simulink model "eqns_motion_mdl_439"  (R2018b)
settings: Solver=VariableStepAuto  StartTime=0.0  StopTime=250  FixedStep=0.1  RelTol=1e-4
values from neighbouring files (symbols this model uses):
  air_data = load('air_data.csv')    [eqns_motion_script.m]    (also in eqns_motion_script_439.m)
  alpha_data = load('alpha_data.csv')    [Test_Runs_Arthur_Function.m]    (also in eqns_motion_script.m; eqns_motion_script_439.m)
  AR = De^2/Dt^2    (= 7.35623218146)    [Test_Runs_Arthur_Function.m]    (also in engineMass.m = engine.output.eql.aeat(3); eqns_motion_script.m = 7.52170654272; eqns_motion_script_439.m = 7.52170654272)
  At = pi*Dt^2/4    (= 7.87496924005)    [Test_Runs_Arthur_Function.m]    (also in engineMass.m = cstar*mdot/(Pc*g); eqns_motion_script.m = 7.53210209316; eqns_motion_script_439.m = 7.53210209316)
  burn_time = (200000+Impulse_Savings)/Thrust    [One_Run.m]    (also in Purdue_Setup.m = 40; Setup.m = 42; Test_Runs.m = 40; Test_Runs_Arthur_Function.m = 39.2156862745)
  Cd_data = load('cd_M.csv')    [Test_Runs_Arthur_Function.m]    (also in eqns_motion_script.m; eqns_motion_script_439.m)
  CG = CG + CG_dot*ts    (= 2.21669239668)    [attempt2.m]    (also in eqns_motion_script.m = 3.6576; eqns_motion_script_439.m = 3.6576; flight_controller.m; flight_sim_3D.m)
  Cn_data = load('cl_M_a.csv')    [Test_Runs_Arthur_Function.m]    (also in eqns_motion_script.m; eqns_motion_script_439.m)
  cp = [CP-CG; 0; 0]    [Y_eqns.m]    (also in Z_eqns.m; attempt2.m; eqns_motion_script.m = 910; eqns_motion_script_439.m = 910)
  Cp_data = load('cp_M_a.csv')    [Test_Runs_Arthur_Function.m]    (also in eqns_motion_script.m; eqns_motion_script_439.m)
  d = D * -v_unit    [Y_eqns.m]    (also in Z_eqns.m; attempt2.m; eqns_motion_script.m = 0.4064; eqns_motion_script_439.m = 0.4064)
  day = 119    [eqns_motion_script.m]    (also in eqns_motion_script_439.m)
  De = 8.5883    [Test_Runs_Arthur_Function.m]    (also in engineMass.m = sqrt(4*Ae/pi); eqns_motion_script.m = 8.4932; eqns_motion_script_439.m = 8.4932)
  h0 = 4595*0.3048    (= 1400.556)    [eqns_motion_script.m]    (also in eqns_motion_script_439.m)
  h_trailer = 75*0.3048    (= 22.86)    [eqns_motion_script.m]    (also in eqns_motion_script_439.m)
  k_he = 0.1177    [eqns_motion_script.m]    (also in eqns_motion_script_439.m)
  kc = 0.35    [eqns_motion_script.m]    (also in eqns_motion_script_439.m)
  lat = 32.9861    [eqns_motion_script.m]    (also in eqns_motion_script_439.m)
  len = 24*0.3048    (= 7.3152)    [attempt2.m]    (also in eqns_motion_script.m; eqns_motion_script_439.m; flight_controller.m; flight_sim_3D.m)
  lon = -106.9717    [eqns_motion_script.m]    (also in eqns_motion_script_439.m)
  M_data = load('M_data.csv')    [Test_Runs_Arthur_Function.m]    (also in eqns_motion_script.m; eqns_motion_script_439.m)
  m_dry = m_dry_lbm / 2.20462    (= 34.0194682077)    [SIM_1DOF.m]    (also in attempt2.m = 330.474171429; eqns_motion_script.m = 291.222339948; eqns_motion_script_439.m = 291.222339948; flight_controller.m = 330.474171429)
  m_wet = 1300*0.453592    (= 589.6696)    [attempt2.m]    (also in eqns_motion_script.m = 679.17690936; eqns_motion_script_439.m = 679.17690936; flight_controller.m; flight_sim_3D.m)
  material_density = 2700    [eqns_motion_script.m]    (also in eqns_motion_script_439.m)
  mdot = mdot + mdot_ffc    [engineMass.m]    (also in eqns_motion_script.m = 10.58683728; eqns_motion_script_439.m = 10.58683728)
  mdot_th = mdot*throttle    (= 10.58683728)    [eqns_motion_script.m]    (also in eqns_motion_script_439.m)
  mu = 1.512041288*(Talt^(3/2))/(Talt+120)    (= 18.1205671028)    [altcond.m]    (also in altcond1.m = 1.512041288*(Talt^(3/2))/(Talt+120); altcond2.m = 1.512041288*(Talt^(3/2))/(Talt+120); eqns_motion_script.m = 0.42; eqns_motion_script_439.m = 0.42)
  Pc = 450    [Test_Runs_Arthur_Function.m]    (also in eqns_motion_script.m; eqns_motion_script_439.m)
  Pe = pressure_integral(end)/burn_time    [Test_Runs.m]    (also in Test_Runs_Arthur_Function.m = 10; eqns_motion_script.m = 10; eqns_motion_script_439.m = 10)
  psi0 = 0    [eqns_motion_script.m]    (also in eqns_motion_script_439.m)
  r = diam/2    (= 0.2286)    [attempt2.m]    (also in eqns_motion_script.m = 0.2032; eqns_motion_script_439.m = 0.2032; flight_controller.m; flight_sim_3D.m)
  sec = 12*3600    (= 43200)    [eqns_motion_script.m]    (also in eqns_motion_script_439.m)
  T = torque_total * 0.113    [PumpSizingModel.m]    (also in attempt2.m = 7000; eqns_motion_script.m = 5100; eqns_motion_script_439.m = 5100; flight_controller.m = 7000)
  t_th = 0    [eqns_motion_script.m]    (also in eqns_motion_script_439.m)
  T_th = T*throttle    (= 5100)    [eqns_motion_script.m]    (also in eqns_motion_script_439.m)
  tc = 0.000    (= 0)    [eqns_motion_script.m]    (also in eqns_motion_script_439.m)
  theta0 = 0    [eqns_motion_script.m]    (also in eqns_motion_script_439.m)
  u0 = 0.1    [eqns_motion_script.m]    (also in eqns_motion_script_439.m)
  v0 = 0.0    (= 0)    [eqns_motion_script.m]    (also in eqns_motion_script_439.m)
  w0 = 0.0    (= 0)    [eqns_motion_script.m]    (also in eqns_motion_script_439.m)
  x = CEA('problem','rocket','equilibrium','o/f', linspace(1,2,5),'p,Mpa',4,'reactants','fuel','N2H4(L)','wt    [CEA.m]    (also in Test_Runs_Arthur_Function.m = 2; eqns_motion_script.m = 0.1; eqns_motion_script_439.m = 0.1; getContour.m = [x_chamber(1:end-1) fliplr(Cx_parabola) x_1_5(2:end) x_0_4(2)
  x1 = len*3/4    (= 5.4864)    [eqns_motion_script.m]    (also in eqns_motion_script_439.m)
libraries: vrlib x8, simulink_extras x6, aerolibutil x3, sharedtransform x2, aerolibasang x2, aerolibconvert2 x2, aerolibatmos2 x1, aerolibadyn x1, aerolibanimutils x1, sharedutil x1, aerolibwind2 x1
settings Model: Creator=Arthur de Waleffe  LastModifiedBy=bartk

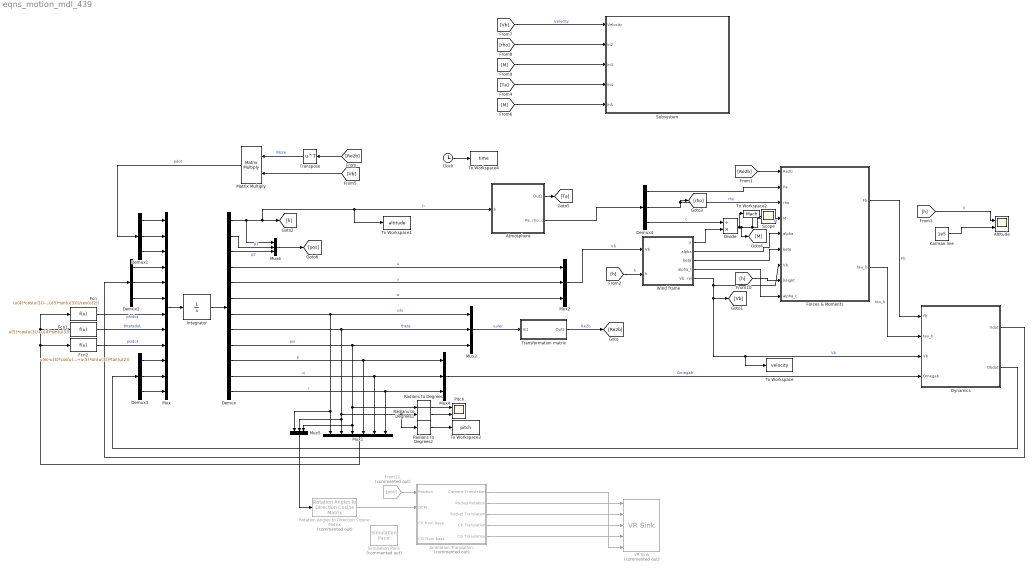
== system eqns_motion_mdl_439 ==
  Altitude : Scope  NumInputPorts=2
  Animation Translation : Subsystem  Commented=on
  Atmosphere : Subsystem
  Clock : Clock
  Demux : Demux  Outputs=12
  Demux{1..4} (4 alike) : Demux  Outputs=3
  Divide : Product  Inputs=/*
  Dynamics : Subsystem
  Fcn : Fcn  Expr=(u(4)*cos(u(3))-u(5)*sin(u(3)))/cos(u(2))
  Fcn1 : Fcn  Expr=u(5)*cos(u(3))+u(4)*sin(u(3))
  Fcn2 : Fcn  Expr=u(6)-u(4)*cos(u(3))*tan(u(2))+u(5)*sin(u(3))*tan(u(2))
  Forces & Moments : Subsystem
  From11 : From  Commented=on  GotoTag=pos
  Integrator : Integrator  InitialCondition=[h0;0;0;u0;v0;w0;0;theta0;psi0;0;0;0]
  Karman line : Constant  Value=1e5
  Matrix Multiply : Product  Multiplication=Matrix(*)
  Mux : Mux  Inputs=12
  Mux1 : Mux  Inputs=6
  Mux{2..6} (5 alike) : Mux  Inputs=3
  Pitch : Scope  NumInputPorts=2
  Radians to Degrees : simulink_extras/Transformations/Radians to Degrees
  Radians to Degrees1 : simulink_extras/Transformations/Radians to Degrees
  Radians to Degrees2 : simulink_extras/Transformations/Radians to Degrees
  Rotation Angles to Direction Cosine Matrix : sharedtransform/Rotation Angles to Direction Cosine Matrix  Commented=on  rotationOrder=ZYX  aMode=aMode
      settings: SourceProductBaseCode=AE
  Scope : Scope
  Simulation Pace : aerolibanimutils/Simulation Pace  Commented=on  SimulationPace=1  SleepMode=Auto  OutputPaceError=off  SampleTime=1/30
  Subsystem : Subsystem
  To Workspace : ToWorkspace  VariableName=velocity  SampleTime=-1
  To Workspace1 : ToWorkspace  VariableName=altitude  SampleTime=-1
  To Workspace2 : ToWorkspace  VariableName=Mach  SaveFormat=Timeseries  SampleTime=-1
  To Workspace3 : ToWorkspace  VariableName=pitch  SaveFormat=Timeseries  SampleTime=-1
  To Workspace4 : ToWorkspace  VariableName=time  SampleTime=-1
  Transformation matrix : Subsystem
  Transpose : Math  Operator=transpose  SaturateOnIntegerOverflow=on
  VR Sink : vrlib/VR Sink  Commented=on  InstantiateOnLoad=on  SampleTime=0.1  ViewEnable=on  RemoteChange=off  RemoteView=off  FieldsWritten=Rocket.rotation.4.1.1.double#Rocket.translation.3.1.1.double#CP.translation.3.1.1.double#CG.translation.3.1.1.double#Camera.position.3.1.1.double  WorldFileName=liftoff.WRL  AutoView=off  VideoDimensions=[]  AllowVariableSize=off
      settings: SourceProductBaseCode=VR
  "Wind frame " : Subsystem
  wires:
  Integrator/1 -> Demux/1
  Mux/1 -> Integrator/1
  Demux/4 -> Mux2/1  "u"
  Demux/5 -> Mux2/2  "v"
  Demux/6 -> Mux2/3  "w"
  Demux/7 -> Mux3/1, Mux5/1, Mux1/1  "phi"
  Demux/8 -> Mux3/2, Radians to Degrees2/1, Radians to Degrees1/1, Mux5/2, Mux1/2  "theta"
  Demux/9 -> Mux3/3, Mux5/3, Mux1/3, Radians to Degrees/1  "psi"
  Demux/10 -> Mux4/1, Mux1/4  "p"
  Demux/12 -> Mux4/3, Mux1/6  "r"
  Demux/11 -> Mux4/2, Mux1/5  "q"
  Fcn/1 -> Mux/7  "phidot"
  Fcn1/1 -> Mux/8  "thtetadot"
  Fcn2/1 -> Mux/9  "psidot"
  Mux1/1 -> Fcn2/1, Fcn/1, Fcn1/1
  Mux3/1 -> Transformation matrix/1(In1)  "euler"
  Transpose/1 -> Matrix Multiply/1  "Rb2e"
  Matrix Multiply/1 -> Demux1/1  "pdot"
  Demux1/2 -> Mux/2
  Demux1/1 -> Mux/1
  Demux1/3 -> Mux/3
  Demux2/1 -> Mux/4
  Demux2/2 -> Mux/5
  Demux2/3 -> Mux/6
  Demux4/2 -> [rho], Forces & Moments/3(rho)  "rho"
  Demux3/1 -> Mux/10
  Demux3/2 -> Mux/11
  Demux3/3 -> Mux/12
  Demux4/3 -> Divide/1  "c"
  Divide/1 -> To Workspace2/1, [M], Scope/1, Forces & Moments/4(M)  "M"
  "Wind frame "/1(V) -> Divide/2
  "Wind frame "/2(alpha) -> Forces & Moments/5(alpha)
  "Wind frame "/3(beta) -> Forces & Moments/6(beta)
  "Wind frame "/4(alpha_t) -> Forces & Moments/9(alpha_t)
  Demux/2 -> Mux6/2  "p1"
  Demux/3 -> Mux6/3  "p2"
  Forces & Moments/1(Fb) -> Dynamics/1(Fb)  "Fb"
  Forces & Moments/2(tau_b) -> Dynamics/2(tau_b)  "tau_b"
  Mux4/1 -> Dynamics/4(Omegab)  "Omegab"
  Dynamics/1(Vdot) -> Demux2/1
  Dynamics/2(Obdot) -> Demux3/1
  Transformation matrix/1(Out1) -> [Re2b]  "Re2b"
  [Re2b] -> Transpose/1
  [Re2b] -> Forces & Moments/1(Re2b)
  [Vb] -> Matrix Multiply/2
  Karman line/1 -> Altitude/2
  [h] -> Altitude/1  "h"
  "Wind frame "/5("Vb, rel") -> [Vb], To Workspace/1, Dynamics/3(Vb), Forces & Moments/7(Vb)  "Vb"
  Mux2/1 -> "Wind frame "/1(Vb)  "Vb"
  Demux4/1 -> Forces & Moments/2(Pa)
  Atmosphere/2("Pa, rho, c") -> Demux4/1
  Demux/1 -> Mux6/1, To Workspace1/1, Atmosphere/1(h), [h]  "h"
  [h] -> "Wind frame "/2(h)  "h"
  [Ta] -> Subsystem/4(In4)
  [M] -> Subsystem/3(In3)
  [Vb] -> Subsystem/1(Velocity)  "Velocity"
  [M] -> Subsystem/5(In5)
  [rho] -> Subsystem/2(In2)
  Atmosphere/1(Out1) -> [Ta]
  [h] -> Forces & Moments/8(height)
  Animation Translation/2(Rocket Rotation) -> VR Sink/1
  Animation Translation/3(Rocket Translation) -> VR Sink/2
  Animation Translation/4(CP Translation) -> VR Sink/3
  Animation Translation/1(Camera Translation) -> VR Sink/5
  Animation Translation/5(CG Translation) -> VR Sink/4
  Mux5/1 -> Rotation Angles to Direction Cosine Matrix/1
  Rotation Angles to Direction Cosine Matrix/1 -> Animation Translation/2(DCM)
  Mux6/1 -> [pos]
  From11/1 -> Animation Translation/1(Position)
  Radians to Degrees/1 -> Pitch/1
  Radians to Degrees1/1 -> Pitch/2
  Radians to Degrees2/1 -> To Workspace3/1
  Clock/1 -> To Workspace4/1

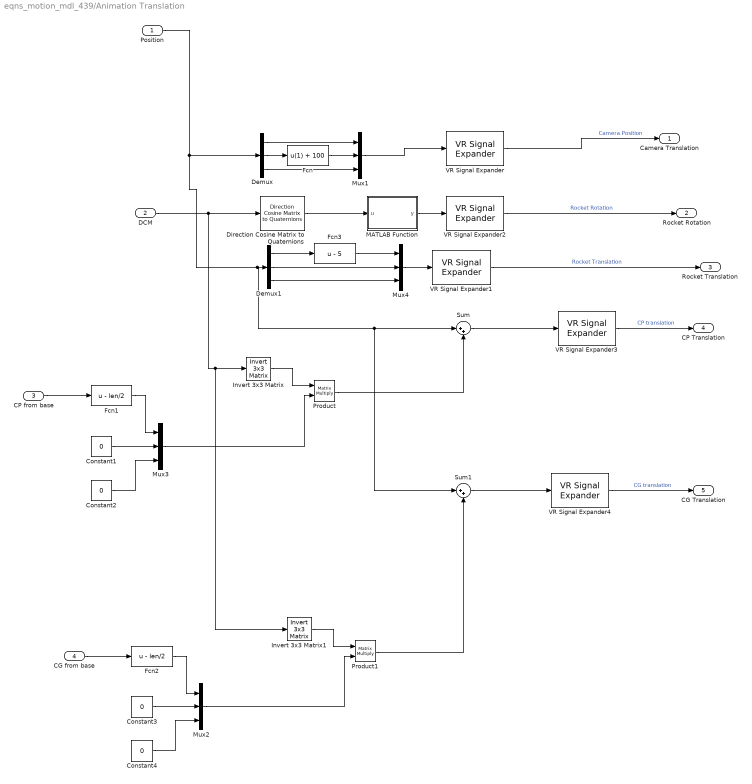
== system eqns_motion_mdl_439/Animation Translation ==
  Position : Inport
  DCM : Inport  Port=2
  CP from base : Inport  Port=3
  CG from base : Inport  Port=4
  Constant{1..4} (4 alike) : Constant  Value=0
  Demux : Demux  Outputs=3
  Demux1 : Demux  Outputs=3
  Direction Cosine Matrix to Quaternions : sharedtransform/Direction Cosine Matrix  to Quaternions  aMode=0  action=None  tolerance=eps(2)
      settings: SourceProductName=Aerospace Blockset  SourceProductBaseCode=AE
  Fcn : Fcn  Expr=u(1) + 100
  Fcn1 : Fcn  Expr=u - len/2
  Fcn2 : Fcn  Expr=u - len/2
  Fcn3 : Fcn  Expr=u - 5
  Invert 3x3 Matrix : aerolibutil/Invert  3x3 Matrix
  Invert 3x3 Matrix1 : aerolibutil/Invert  3x3 Matrix
  MATLAB Function : MATLAB Function  TreatAsAtomicUnit=on
  Mux{1..4} (4 alike) : Mux  Inputs=3
  Product : Product  Multiplication=Matrix(*)
  Product1 : Product  Multiplication=Matrix(*)
  Sum : Sum  Inputs=|++
  Sum1 : Sum  Inputs=|++
  VR Signal Expander{,1,3..4} (4 alike) : vrlib/VR Signal Expander  outwidth=3  outidx=[2 3 1]
      settings: SourceProductName=Simulink 3D Animation  SourceProductBaseCode=VR
  VR Signal Expander2 : vrlib/VR Signal Expander  outwidth=4  outidx=[2 3 1 4]
      settings: SourceProductName=Simulink 3D Animation  SourceProductBaseCode=VR
  Camera Translation : Outport
  Rocket Rotation : Outport  Port=2
  Rocket Translation : Outport  Port=3
  CP Translation : Outport  Port=4
  CG Translation : Outport  Port=5
  wires:
  Demux/2 -> Fcn/1
  Position/1 -> Demux1/1, Sum1/1, Sum/1, Demux/1
  Mux1/1 -> VR Signal Expander/1
  MATLAB Function/1(y) -> VR Signal Expander2/1
  DCM/1 -> Invert 3x3 Matrix1/1, Invert 3x3 Matrix/1, Direction Cosine Matrix to Quaternions/1
  Direction Cosine Matrix to Quaternions/1 -> MATLAB Function/1(u)
  Demux/3 -> Mux1/3
  Demux/1 -> Mux1/1
  Fcn/1 -> Mux1/2
  VR Signal Expander/1 -> Camera Translation/1  "Camera Position"
  CP from base/1 -> Fcn1/1
  VR Signal Expander3/1 -> CP Translation/1  "CP translation"
  Constant1/1 -> Mux3/2
  Fcn1/1 -> Mux3/1
  Constant2/1 -> Mux3/3
  Mux3/1 -> Product/2
  Product/1 -> Sum/2
  Invert 3x3 Matrix/1 -> Product/1
  Sum/1 -> VR Signal Expander3/1
  VR Signal Expander2/1 -> Rocket Rotation/1  "Rocket Rotation"
  VR Signal Expander1/1 -> Rocket Translation/1  "Rocket Translation"
  Constant4/1 -> Mux2/3
  Invert 3x3 Matrix1/1 -> Product1/1
  Mux2/1 -> Product1/2
  Fcn2/1 -> Mux2/1
  Constant3/1 -> Mux2/2
  CG from base/1 -> Fcn2/1
  Product1/1 -> Sum1/2
  Sum1/1 -> VR Signal Expander4/1
  VR Signal Expander4/1 -> CG Translation/1  "CG translation"
  Demux1/3 -> Mux4/3
  Demux1/2 -> Mux4/2
  Mux4/1 -> VR Signal Expander1/1
  Demux1/1 -> Fcn3/1
  Fcn3/1 -> Mux4/1

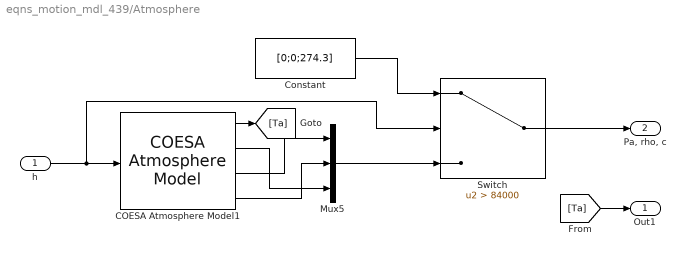
== system eqns_motion_mdl_439/Atmosphere ==
  h : Inport
  COESA Atmosphere Model1 : aerolibatmos2/COESA Atmosphere Model  units=Metric (MKS)  spec=1976 COESA-extended U.S. Standard Atmosphere  model=Profile  profile_var=High temperature  profile_percent=1%  profile_alt=5 km (16404 ft)  envelope_var=High temperature  envelope_percent=1%  action=Warning
  Constant : Constant  Value=[0;0;274.3]
  Mux5 : Mux  Inputs=3
  Switch : Switch  Criteria=u2 > Threshold  Threshold=84000
  Out1 : Outport
  "Pa, rho, c" : Outport  Port=2
  wires:
  Switch/1 -> "Pa, rho, c"/1
  COESA Atmosphere Model1/3 -> Mux5/1
  Constant/1 -> Switch/1
  Mux5/1 -> Switch/3
  COESA Atmosphere Model1/1 -> [Ta]
  COESA Atmosphere Model1/4 -> Mux5/2
  COESA Atmosphere Model1/2 -> Mux5/3
  h/1 -> COESA Atmosphere Model1/1, Switch/2
  [Ta] -> Out1/1

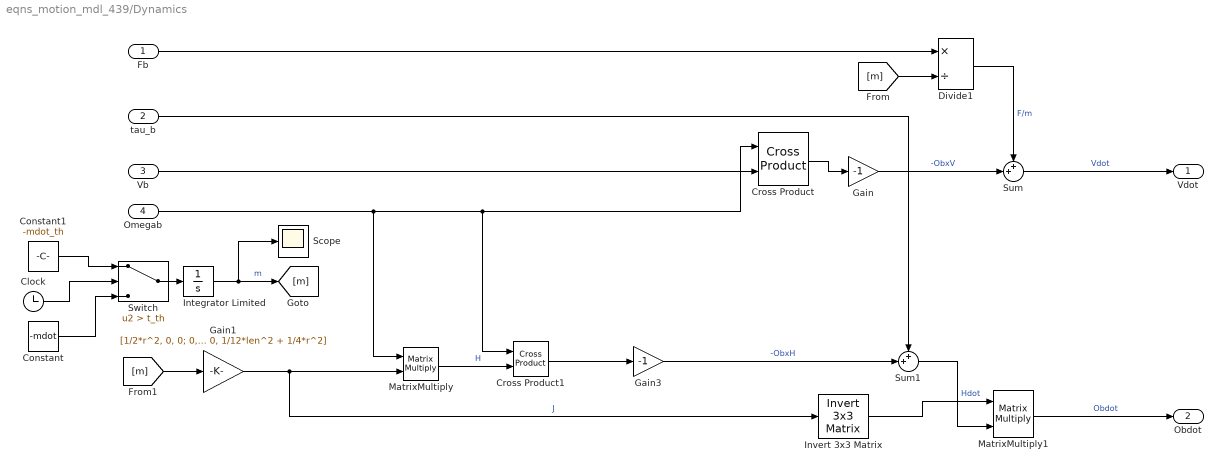
== system eqns_motion_mdl_439/Dynamics ==
  Fb : Inport
  tau_b : Inport  Port=2
  Vb : Inport  Port=3
  Omegab : Inport  Port=4
  Clock : Clock
  Constant : Constant  Value=-mdot
  Constant1 : Constant  Value=-mdot_th
  Cross Product : vrlib/Utilities/Cross Product
      settings: SourceProductBaseCode=VR
  Cross Product1 : vrlib/Utilities/Cross Product
      settings: SourceProductBaseCode=VR
  Divide1 : Product  Inputs=*/
  Gain : Gain  Gain=-1
  Gain1 : Gain  Gain=[1/2*r^2, 0, 0; 0, 1/12*len^2 + 1/4*r^2, 0; 0, 0, 1/12*len^2 + 1/4*r^2]
  Gain3 : Gain  Gain=-1
  Integrator Limited : Integrator  InitialCondition=m_wet  LimitOutput=on  UpperSaturationLimit=m_wet  LowerSaturationLimit=m_dry
  Invert 3x3 Matrix : aerolibutil/Invert  3x3 Matrix
  MatrixMultiply : Product  Multiplication=Matrix(*)
  MatrixMultiply1 : Product  Multiplication=Matrix(*)
  Scope : Scope
  Sum : Sum  Inputs=++|
  Sum1 : Sum  Inputs=++|
  Switch : Switch  Criteria=u2 > Threshold  Threshold=t_th
  Vdot : Outport
  Obdot : Outport  Port=2
  wires:
  Gain1/1 -> Invert 3x3 Matrix/1, MatrixMultiply/2  "J"
  MatrixMultiply/1 -> Cross Product1/2  "H"
  MatrixMultiply1/1 -> Obdot/1  "Obdot"
  Cross Product/1 -> Gain/1
  Sum1/1 -> MatrixMultiply1/2  "Hdot"
  Integrator Limited/1 -> Scope/1, [m]  "m"
  Gain3/1 -> Sum1/2  "-ObxH"
  Cross Product1/1 -> Gain3/1
  Omegab/1 -> Cross Product/1, Cross Product1/1, MatrixMultiply/1
  Gain/1 -> Sum/2  "-ObxV"
  Invert 3x3 Matrix/1 -> MatrixMultiply1/1
  Sum/1 -> Vdot/1  "Vdot"
  Divide1/1 -> Sum/1  "F/m"
  Vb/1 -> Cross Product/2
  Fb/1 -> Divide1/1
  tau_b/1 -> Sum1/1
  [m] -> Divide1/2
  [m] -> Gain1/1
  Clock/1 -> Switch/2
  Constant1/1 -> Switch/1
  Constant/1 -> Switch/3
  Switch/1 -> Integrator Limited/1

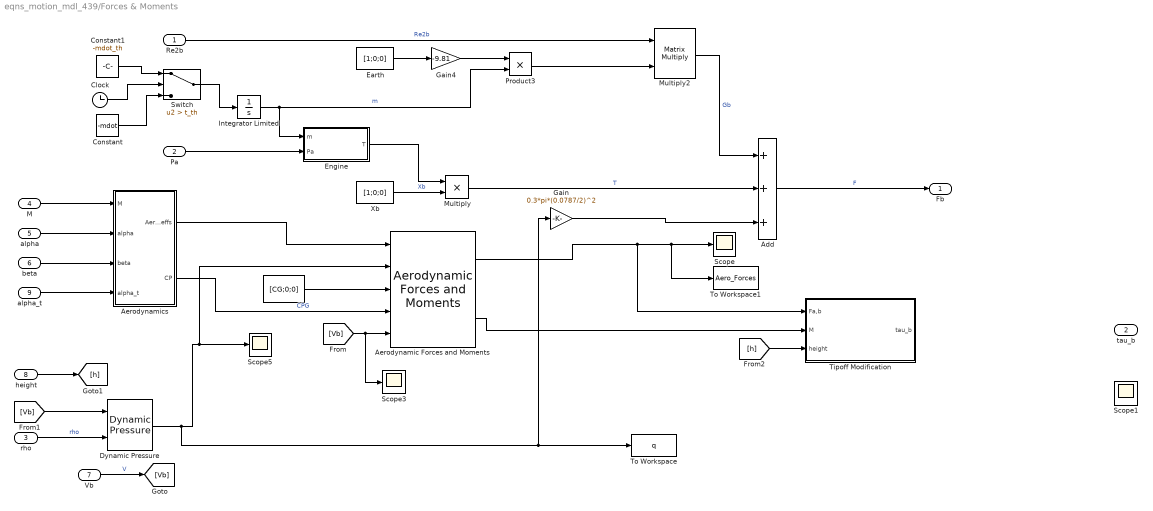
== system eqns_motion_mdl_439/Forces & Moments ==
  Re2b : Inport
  Pa : Inport  Port=2
  rho : Inport  Port=3
  M : Inport  Port=4
  alpha : Inport  Port=5
  beta : Inport  Port=6
  Vb : Inport  Port=7
  height : Inport  Port=8
  alpha_t : Inport  Port=9
  " " : Constant  Value=[CG;0;0]
  Add : Sum  Inputs=+++
  "Aerodynamic Forces and Moments " : aerolibadyn/Aerodynamic Forces and Moments   inputAxes=Wind  outputForceAxes=Body  outputMomentAxes=Body  S=S  b=d  cbar=len
      settings: SourceProductName=Aerospace Blockset
  Aerodynamics : Subsystem
  Clock : Clock
  Constant : Constant  Value=-mdot
  Constant1 : Constant  Value=-mdot_th
  Dynamic Pressure : aerolibasang/Dynamic Pressure
  Earth : Constant  Value=[1;0;0]
  Engine : Subsystem
  Gain : Gain  Gain=0.3*pi*(0.0787/2)^2
  Gain4 : Gain  Gain=-9.81
  Integrator Limited : Integrator  InitialCondition=m_wet  LimitOutput=on  UpperSaturationLimit=m_wet  LowerSaturationLimit=m_dry
  Multiply : Product
  Multiply2 : Product  Multiplication=Matrix(*)
  Product3 : Product
  Scope{,1,3,5} (4 alike) : Scope
  Switch : Switch  Criteria=u2 > Threshold  Threshold=t_th
  Tipoff Modification : Subsystem
  To Workspace : ToWorkspace  VariableName=q  SaveFormat=Timeseries  SampleTime=-1
  To Workspace1 : ToWorkspace  VariableName=Aero_Forces  SaveFormat=Timeseries  SampleTime=-1
  Xb : Constant  Value=[1;0;0]
  Fb : Outport
  tau_b : Outport  Port=2
  wires:
  Multiply2/1 -> Add/1  "Gb"
  Re2b/1 -> Multiply2/1  "Re2b"
  Earth/1 -> Gain4/1
  Add/1 -> Fb/1  "F"
  Gain4/1 -> Product3/1
  Integrator Limited/1 -> Engine/1(m), Product3/2  "m"
  Product3/1 -> Multiply2/2
  Xb/1 -> Multiply/2  "Xb"
  Multiply/1 -> Add/2  "T"
  rho/1 -> Dynamic Pressure/2  "rho"
  Aerodynamics/1(Aero coeffs) -> "Aerodynamic Forces and Moments "/1
  Aerodynamics/2(CP) -> "Aerodynamic Forces and Moments "/4  "CPG"
  " "/1 -> "Aerodynamic Forces and Moments "/3
  [Vb] -> Scope3/1, "Aerodynamic Forces and Moments "/5
  [Vb] -> Dynamic Pressure/1
  Pa/1 -> Engine/2(Pa)
  Engine/1(T) -> Multiply/1
  Switch/1 -> Integrator Limited/1
  Constant/1 -> Switch/3
  Constant1/1 -> Switch/1
  Clock/1 -> Switch/2
  [h] -> Tipoff Modification/3(height)
  "Aerodynamic Forces and Moments "/2 -> Tipoff Modification/2(M)
  "Aerodynamic Forces and Moments "/1 -> Tipoff Modification/1(Fa,b), To Workspace1/1, Scope/1
  height/1 -> [h]
  Vb/1 -> [Vb]  "V"
  alpha/1 -> Aerodynamics/2(alpha)
  beta/1 -> Aerodynamics/3(beta)
  M/1 -> Aerodynamics/1(M)
  Dynamic Pressure/1 -> Gain/1, To Workspace/1, Scope5/1, "Aerodynamic Forces and Moments "/2
  alpha_t/1 -> Aerodynamics/4(alpha_t)
  Gain/1 -> Add/3

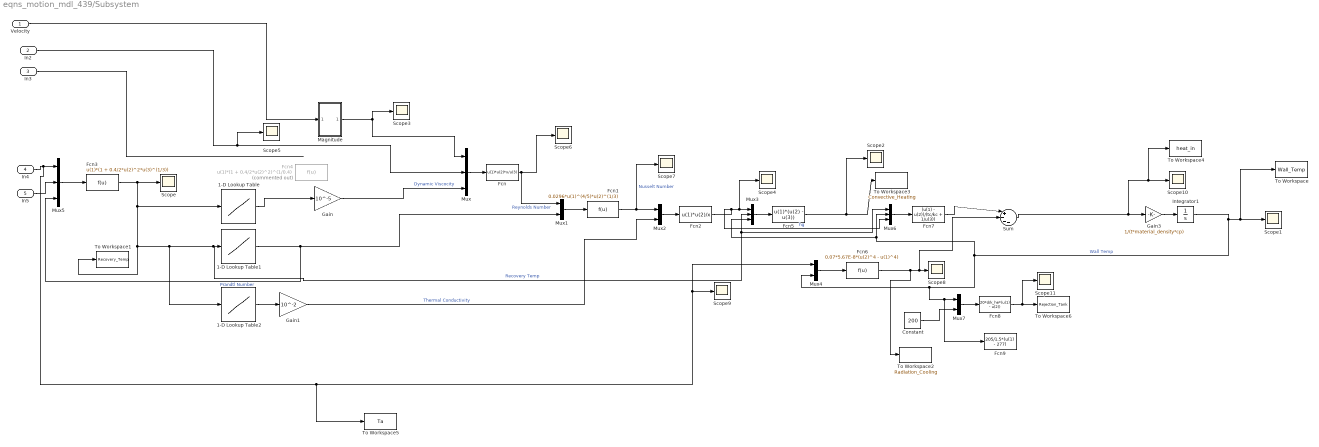
== system eqns_motion_mdl_439/Subsystem ==
  Velocity : Inport
  In2 : Inport  Port=2
  In3 : Inport  Port=3
  In4 : Inport  Port=4
  In5 : Inport  Port=5
  1-D Lookup Table : Lookup_n-D  NumberOfTableDimensions=1  BreakpointsForDimension1=air_data(:,1)  Table=air_data(:,5)  InternalRulePriority=Speed  RndMeth=Simplest  InputSameDT=on
  1-D Lookup Table1 : Lookup_n-D  NumberOfTableDimensions=1  BreakpointsForDimension1=air_data(:,1)  Table=air_data(:,7)  InternalRulePriority=Speed  RndMeth=Simplest  InputSameDT=on
  1-D Lookup Table2 : Lookup_n-D  NumberOfTableDimensions=1  BreakpointsForDimension1=air_data(:,1)  Table=air_data(:,6)  InternalRulePriority=Speed  RndMeth=Simplest  InputSameDT=on
  Constant : Constant  Value=200
  Fcn : Fcn  Expr=u(1)*u(2)*x/u(3)
  Fcn1 : Fcn  Expr=0.0296*u(1)^(4/5)*u(2)^(1/3)
  Fcn2 : Fcn  Expr=u(1)*u(2)/x
  Fcn3 : Fcn  Expr=u(1)*(1 + 0.4/2*u(2)^2*u(3)^(1/3))
  Fcn4 : Fcn  Commented=on  Expr=u(1)*(1 + 0.4/2*u(2)^2)^(1/0.4)
  Fcn5 : Fcn  Expr=u(1)*(u(2) - u(3))
  Fcn6 : Fcn  Expr=0.07*5.67E-8*(u(2)^4 - u(1)^4)
  Fcn7 : Fcn  Expr=(u(1) - u(2))/(tc/kc + 1/u(3))
  Fcn8 : Fcn  Expr=20*d/k_he*(u(1) - u(2))
  Fcn9 : Fcn  Expr=205/1.5*(u(1) - 277)
  Gain : Gain  Gain=10^-5
  Gain1 : Gain  Gain=10^-2
  Gain3 : Gain  Gain=1/(t*material_density*cp)
  Integrator1 : Integrator  InitialCondition=277
  Magnitude : Subsystem
  Mux{,3,5..6} (4 alike) : Mux  Inputs=3
  Mux{1..2,4,7} (4 alike) : Mux  Inputs=2
  Scope{,1..11} (12 alike) : Scope
  Sum : Sum  Inputs=|+---
  To Workspace : ToWorkspace  VariableName=Wall_Temp  SaveFormat=Timeseries  SampleTime=-1
  To Workspace1 : ToWorkspace  VariableName=Recovery_Temp  SaveFormat=Timeseries  SampleTime=-1
  To Workspace2 : ToWorkspace  VariableName=Radiation_Cooling  SaveFormat=Timeseries  SampleTime=-1
  To Workspace3 : ToWorkspace  VariableName=Convective_Heating  SaveFormat=Timeseries  SampleTime=-1
  To Workspace4 : ToWorkspace  VariableName=heat_in  SaveFormat=Structure With Time  SampleTime=-1
  To Workspace5 : ToWorkspace  VariableName=Ta  SaveFormat=Timeseries  SampleTime=-1
  To Workspace6 : ToWorkspace  VariableName=Rejection_Tank  SaveFormat=Timeseries  SampleTime=-1
  wires:
  Gain1/1 -> Mux2/2  "Thermal Conductivity"
  Mux5/1 -> Fcn3/1
  Fcn3/1 -> To Workspace1/1, 1-D Lookup Table2/1, Mux6/1, Mux3/2, 1-D Lookup Table1/1, 1-D Lookup Table/1, Scope/1  "Recovery Temp"
  1-D Lookup Table1/1 -> Mux1/2, Mux5/3  "Prandtl Number"
  In2/1 -> Mux/2, Scope5/1
  In3/1 -> ?
  1-D Lookup Table2/1 -> Gain1/1
  Gain/1 -> Mux/3  "Dynamic Viscocity"
  Integrator1/1 -> Mux6/2, Mux3/3, Fcn9/1, Mux7/1, Mux4/2, To Workspace/1, Scope1/1  "Wall Temp"
  In5/1 -> Mux5/2
  Magnitude/1(Out1) -> Mux/1, Scope3/1
  1-D Lookup Table/1 -> Gain/1
  Velocity/1 -> Magnitude/1(Velocity)
  In4/1 -> To Workspace5/1, Scope9/1, Mux4/1, Mux5/1
  Mux/1 -> Fcn/1
  Fcn/1 -> Mux1/1, Scope6/1  "Reynolds Number"
  Mux1/1 -> Fcn1/1
  Fcn1/1 -> Scope7/1, Mux2/1  "Nusselt Number"
  Mux2/1 -> Fcn2/1
  Fcn2/1 -> Scope4/1, Mux3/1, Mux6/3  "hg"
  Mux3/1 -> Fcn5/1
  Fcn5/1 -> Scope2/1, To Workspace3/1
  Fcn6/1 -> To Workspace2/1, Sum/2, Scope8/1
  Mux4/1 -> Fcn6/1
  Gain3/1 -> Integrator1/1
  Fcn7/1 -> Sum/1
  Mux6/1 -> Fcn7/1
  Constant/1 -> Mux7/2
  Mux7/1 -> Fcn8/1
  Fcn8/1 -> Scope11/1, To Workspace6/1
  Sum/1 -> To Workspace4/1, Scope10/1, Gain3/1

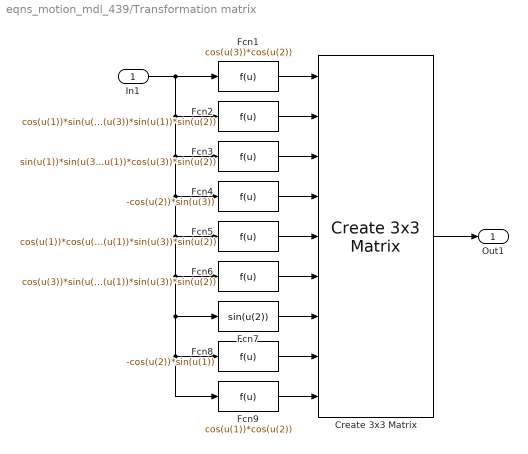
== system eqns_motion_mdl_439/Transformation matrix ==
  In1 : Inport
  Create 3x3 Matrix : sharedutil/Create 3x3 Matrix  aMode=aMode
  Fcn1 : Fcn  Expr=cos(u(3))*cos(u(2))
  Fcn2 : Fcn  Expr=cos(u(1))*sin(u(3)) + cos(u(3))*sin(u(1))*sin(u(2))
  Fcn3 : Fcn  Expr=sin(u(1))*sin(u(3)) - cos(u(1))*cos(u(3))*sin(u(2))
  Fcn4 : Fcn  Expr=-cos(u(2))*sin(u(3))
  Fcn5 : Fcn  Expr=cos(u(1))*cos(u(3)) - sin(u(1))*sin(u(3))*sin(u(2))
  Fcn6 : Fcn  Expr=cos(u(3))*sin(u(1)) + cos(u(1))*sin(u(3))*sin(u(2))
  Fcn7 : Fcn  Expr=sin(u(2))
  Fcn8 : Fcn  Expr=-cos(u(2))*sin(u(1))
  Fcn9 : Fcn  Expr=cos(u(1))*cos(u(2))
  Out1 : Outport
  wires:
  In1/1 -> Fcn9/1, Fcn8/1, Fcn7/1, Fcn6/1, Fcn5/1, Fcn4/1, Fcn3/1, Fcn2/1, Fcn1/1
  Fcn9/1 -> Create 3x3 Matrix/9
  Fcn8/1 -> Create 3x3 Matrix/8
  Fcn7/1 -> Create 3x3 Matrix/7
  Fcn6/1 -> Create 3x3 Matrix/6
  Fcn5/1 -> Create 3x3 Matrix/5
  Fcn4/1 -> Create 3x3 Matrix/4
  Fcn3/1 -> Create 3x3 Matrix/3
  Fcn2/1 -> Create 3x3 Matrix/2
  Fcn1/1 -> Create 3x3 Matrix/1
  Create 3x3 Matrix/1 -> Out1/1

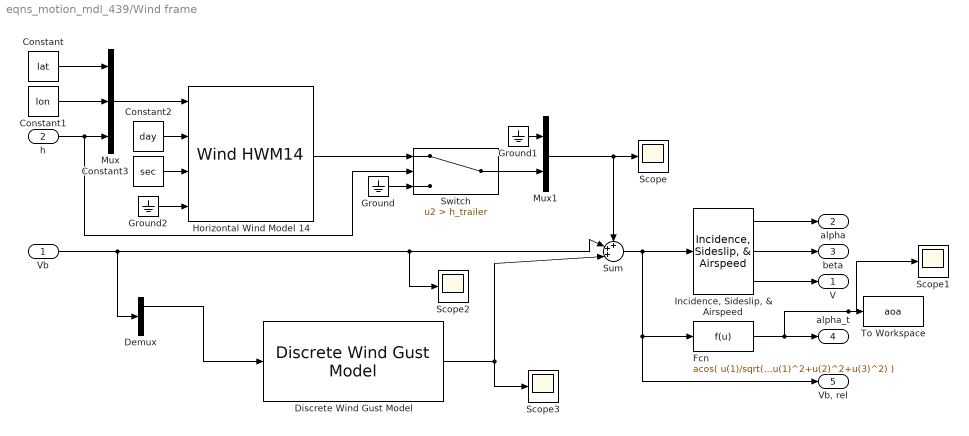
== system eqns_motion_mdl_439/Wind frame  ==
  Vb : Inport
  h : Inport  Port=2
  Constant : Constant  Value=lat
  Constant1 : Constant  Value=lon
  Constant2 : Constant  Value=day
  Constant3 : Constant  Value=sec
  Demux : Demux  Outputs=3
  Discrete Wind Gust Model : aerolibwind2/Discrete Wind Gust Model  units=Metric (MKS)  Gx=on  Gy=on  Gz=on  t_0=20  d_m=[100 100 100]  v_m=[0 0 0]
      settings: SourceProductName=Aerospace Blockset
  Fcn : Fcn  Expr=acos( u(1)/sqrt(u(1)^2+u(2)^2+u(3)^2) )
  Ground : Ground
  Ground1 : Ground
  Ground2 : Ground
  Horizontal Wind Model 14 : WindHWM14  model=Total
  "Incidence, Sideslip, & Airspeed" : aerolibasang/Incidence, Sideslip, & Airspeed
      settings: SourceProductName=Aerospace Blockset
  Mux : Mux  Inputs=3
  Mux1 : Mux  Inputs=2
  Scope{,1..3} (4 alike) : Scope
  Sum : Sum  Inputs=+++|
  Switch : Switch  Criteria=u2 > Threshold  Threshold=h_trailer
  To Workspace : ToWorkspace  VariableName=aoa  SaveFormat=Timeseries  SampleTime=-1
  V : Outport
  alpha : Outport  Port=2
  beta : Outport  Port=3
  alpha_t : Outport  Port=4
  "Vb, rel" : Outport  Port=5
  wires:
  Sum/1 -> "Vb, rel"/1, Fcn/1, "Incidence, Sideslip, & Airspeed"/1
  "Incidence, Sideslip, & Airspeed"/3 -> V/1
  "Incidence, Sideslip, & Airspeed"/1 -> alpha/1
  "Incidence, Sideslip, & Airspeed"/2 -> beta/1
  Fcn/1 -> Scope1/1, To Workspace/1, alpha_t/1
  h/1 -> Switch/2, Mux/3
  Mux/1 -> Horizontal Wind Model 14/1
  Constant1/1 -> Mux/2
  Constant/1 -> Mux/1
  Constant2/1 -> Horizontal Wind Model 14/2
  Constant3/1 -> Horizontal Wind Model 14/3
  Horizontal Wind Model 14/1 -> Switch/1
  Ground/1 -> Switch/3
  Switch/1 -> Mux1/2
  Ground1/1 -> Mux1/1
  Vb/1 -> Demux/1, Scope2/1, Sum/2
  Ground2/1 -> Horizontal Wind Model 14/4
  Mux1/1 -> Sum/1, Scope/1
  Discrete Wind Gust Model/1 -> Scope3/1, Sum/3
  Demux/1 -> Discrete Wind Gust Model/1

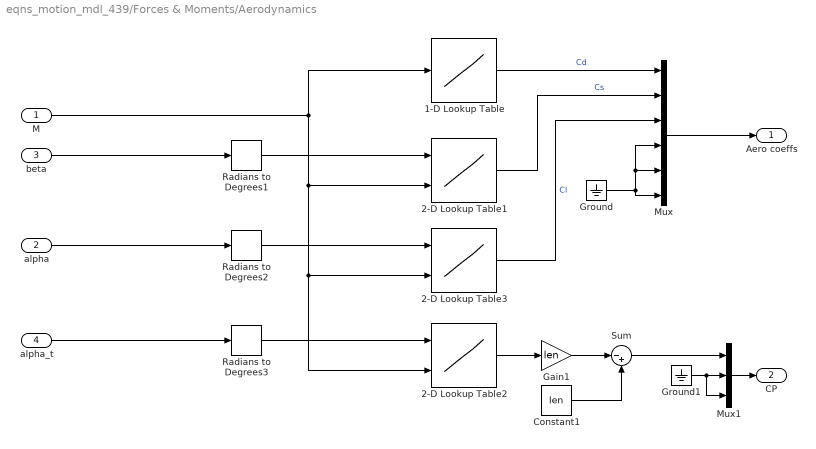
== system eqns_motion_mdl_439/Forces & Moments/Aerodynamics ==
  M : Inport
  alpha : Inport  Port=2
  beta : Inport  Port=3
  alpha_t : Inport  Port=4
  1-D Lookup Table : Lookup_n-D  NumberOfTableDimensions=1  BreakpointsForDimension1=M_data  Table=Cd_data  InternalRulePriority=Speed  RndMeth=Simplest  InputSameDT=on
  2-D Lookup Table1 : Lookup_n-D  BreakpointsForDimension1=alpha_data  BreakpointsForDimension2=M_data  Table=Cn_data  InternalRulePriority=Speed  RndMeth=Simplest  InputSameDT=on
  2-D Lookup Table2 : Lookup_n-D  BreakpointsForDimension1=alpha_data  BreakpointsForDimension2=M_data  Table=Cp_data  InternalRulePriority=Speed  RndMeth=Simplest  InputSameDT=on
  2-D Lookup Table3 : Lookup_n-D  BreakpointsForDimension1=alpha_data  BreakpointsForDimension2=M_data  Table=Cn_data  InternalRulePriority=Speed  RndMeth=Simplest  InputSameDT=on
  Constant1 : Constant  Value=len  VectorParams1D=off
  Gain1 : Gain  Gain=len
  Ground : Ground
  Ground1 : Ground
  Mux : Mux  Inputs=6
  Mux1 : Mux  Inputs=3
  Radians to Degrees1 : simulink_extras/Transformations/Radians to Degrees
  Radians to Degrees2 : simulink_extras/Transformations/Radians to Degrees
  Radians to Degrees3 : simulink_extras/Transformations/Radians to Degrees
  Sum : Sum  Inputs=|-+
  Aero coeffs : Outport
  CP : Outport  Port=2
  wires:
  1-D Lookup Table/1 -> Mux/1  "Cd"
  2-D Lookup Table2/1 -> Gain1/1
  2-D Lookup Table1/1 -> Mux/2  "Cs"
  2-D Lookup Table3/1 -> Mux/3  "Cl"
  beta/1 -> Radians to Degrees1/1
  alpha/1 -> Radians to Degrees2/1
  M/1 -> 2-D Lookup Table1/2, 2-D Lookup Table2/2, 2-D Lookup Table3/2, 1-D Lookup Table/1
  Radians to Degrees1/1 -> 2-D Lookup Table1/1
  Radians to Degrees2/1 -> 2-D Lookup Table3/1
  alpha_t/1 -> Radians to Degrees3/1
  Radians to Degrees3/1 -> 2-D Lookup Table2/1
  Ground/1 -> Mux/4, Mux/5, Mux/6
  Mux/1 -> Aero coeffs/1
  Gain1/1 -> Sum/1
  Constant1/1 -> Sum/2
  Sum/1 -> Mux1/1
  Mux1/1 -> CP/1
  Ground1/1 -> Mux1/2, Mux1/3

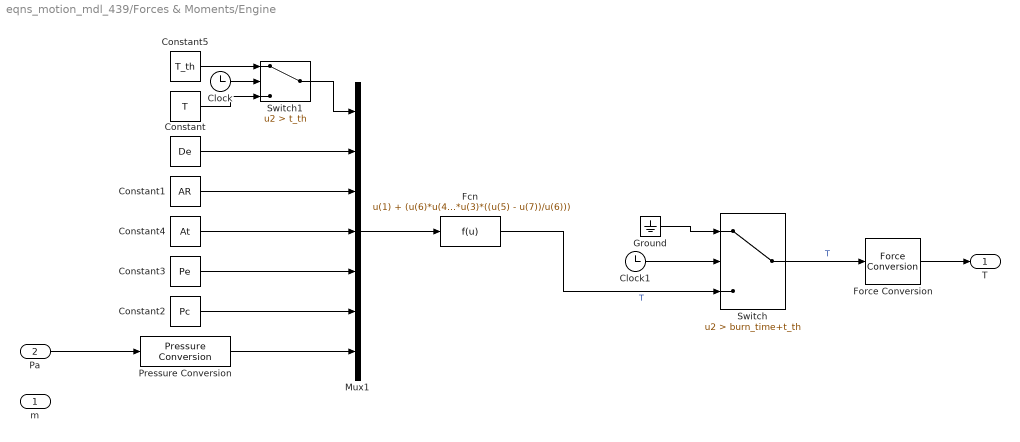
== system eqns_motion_mdl_439/Forces & Moments/Engine ==
  m : Inport
  Pa : Inport  Port=2
  " " : Constant  Value=T
  Clock : Clock
  Clock1 : Clock
  Constant : Constant  Value=De
  Constant1 : Constant  Value=AR
  Constant2 : Constant  Value=Pc
  Constant3 : Constant  Value=Pe
  Constant4 : Constant  Value=At
  Constant5 : Constant  Value=T_th
  Fcn : Fcn  Expr=u(1) + (u(6)*u(4)*u(3)*((u(5) - u(7))/u(6)))
  Force Conversion : aerolibconvert2/Force Conversion  IU=lbf  OU=N
      settings: SourceProductName=Aerospace Blockset  SourceProductBaseCode=AE
  Ground : Ground
  Mux1 : Mux  Inputs=7
  Pressure Conversion : aerolibconvert2/Pressure Conversion  IU=Pa  OU=psi
      settings: SourceProductName=Aerospace Blockset  SourceProductBaseCode=AE
  Switch : Switch  Criteria=u2 > Threshold  Threshold=burn_time+t_th
  Switch1 : Switch  Criteria=u2 > Threshold  Threshold=t_th
  T : Outport
  wires:
  Constant2/1 -> Mux1/6
  Constant3/1 -> Mux1/5
  Mux1/1 -> Fcn/1
  Constant1/1 -> Mux1/3
  Constant/1 -> Mux1/2
  Pa/1 -> Pressure Conversion/1
  Constant4/1 -> Mux1/4
  Switch/1 -> Force Conversion/1  "T"
  Force Conversion/1 -> T/1
  Pressure Conversion/1 -> Mux1/7
  Constant5/1 -> Switch1/1
  " "/1 -> Switch1/3
  Clock/1 -> Switch1/2
  Switch1/1 -> Mux1/1
  Clock1/1 -> Switch/2
  Ground/1 -> Switch/1
  Fcn/1 -> Switch/3  "T"

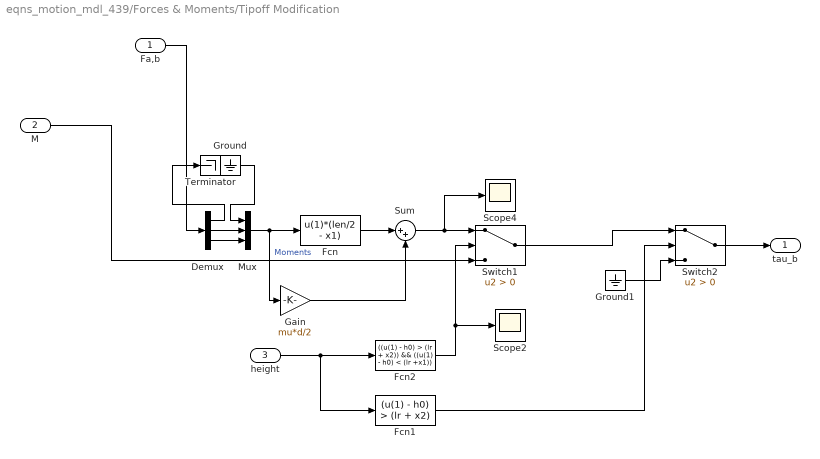
== system eqns_motion_mdl_439/Forces & Moments/Tipoff Modification ==
  Fa,b : Inport
  M : Inport  Port=2
  height : Inport  Port=3
  Demux : Demux  Outputs=3
  Fcn : Fcn  Expr=u(1)*(len/2 - x1)
  Fcn1 : Fcn  Expr=(u(1) - h0) > (lr + x2)
  Fcn2 : Fcn  Expr=((u(1) - h0) > (lr + x2)) && ((u(1) - h0) < (lr +x1))
  Gain : Gain  Gain=mu*d/2
  Ground : Ground
  Ground1 : Ground
  Mux : Mux  Inputs=3
  Scope2 : Scope
  Scope4 : Scope
  Sum : Sum  Inputs=|++
  Switch1 : Switch  Criteria=u2 > Threshold
  Switch2 : Switch  Criteria=u2 > Threshold
  Terminator : Terminator
  tau_b : Outport
  wires:
  height/1 -> Fcn1/1, Fcn2/1
  Gain/1 -> Sum/2
  Switch1/1 -> Switch2/1
  Sum/1 -> Scope4/1, Switch1/1
  Fcn/1 -> Sum/1
  Fcn1/1 -> Switch2/2
  Ground/1 -> Mux/1
  M/1 -> Switch1/3  "Moments"
  Demux/1 -> Terminator/1
  Demux/3 -> Mux/3
  Mux/1 -> Gain/1, Fcn/1
  Switch2/1 -> tau_b/1
  Demux/2 -> Mux/2
  Ground1/1 -> Switch2/3
  Fa,b/1 -> Demux/1
  Fcn2/1 -> Switch1/2, Scope2/1

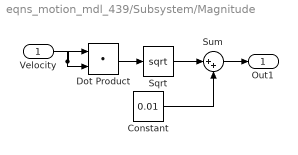
== system eqns_motion_mdl_439/Subsystem/Magnitude ==
  Velocity : Inport
  Constant : Constant  Value=0.01
  Dot Product : DotProduct  InputSameDT=on  OutDataTypeStr=Inherit: Inherit via internal rule
  Sqrt : Sqrt  SaturateOnIntegerOverflow=on
  Sum : Sum  Inputs=|++
  Out1 : Outport
  wires:
  Sum/1 -> Out1/1
  Velocity/1 -> Dot Product/2, Dot Product/1
  Dot Product/1 -> Sqrt/1
  Constant/1 -> Sum/2
  Sqrt/1 -> Sum/1

== matlab function eqns_motion_mdl_439/Animation Translation/MATLAB Function ==
  data: u input; y output
function y = fcn(u)
y = [0; 0; 0; 0];
y(1) = u(2)/sqrt(1-u(1)^2);
y(2) = u(3)/sqrt(1-u(1)^2);
y(3) = u(4)/sqrt(1-u(1)^2);
y(4) = 2 * acos(u(1));
end
